simulink model "dis_lin"  (R2020b)
settings: Solver=VariableStepAuto  StartTime=0.0  StopTime=50.0  RelTol=1e-3
values from neighbouring files (symbols this model uses):
  alpha = 0.95    [main.m]
  amp = 0.3    [main.m]
  Ts = 0.15    [main.m]
  x_equ = [0.2; 0]    [main.m]
settings Model: Creator=soren  LastModifiedBy=soren

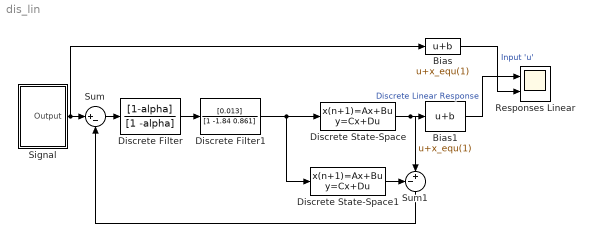
== system dis_lin ==
  Bias : Bias  Bias=x_equ(1)
  Bias1 : Bias  Bias=x_equ(1)
  Discrete Filter : DiscreteFilter  Numerator=[1-alpha]  Denominator=[1 -alpha]
  Discrete Filter1 : DiscreteFilter  Numerator=[0.013]  Denominator=[1 -1.84 0.861]
  Discrete State-Space : DiscreteStateSpace  A=[1 Ts;-3/4*Ts 1-Ts]  B=[0; 1.25*Ts]  C=[1, 0]  D=0  SampleTime=Ts
  Discrete State-Space1 : DiscreteStateSpace  A=[1 Ts;-3/4*Ts 1-Ts]  B=[0; 1.25*Ts]  C=[1, 0]  D=0  SampleTime=Ts
  Responses Linear : Scope  NumInputPorts=2
  Signal : Subsystem
  Sum : Sum  Inputs=|+-
  Sum1 : Sum  Inputs=-+|
  wires:
  Signal/1(Output) -> Bias/1, Sum/1
  Discrete Filter/1 -> Discrete Filter1/1
  Sum/1 -> Discrete Filter/1
  Discrete State-Space/1 -> Bias1/1, Sum1/2
  Discrete Filter1/1 -> Discrete State-Space1/1, Discrete State-Space/1
  Sum1/1 -> Sum/2
  Bias1/1 -> Responses Linear/1  "Discrete Linear Response"
  Bias/1 -> Responses Linear/2  "Input 'u'"
  Discrete State-Space1/1 -> Sum1/1

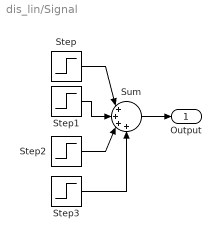
== system dis_lin/Signal ==
  Step : Step  Time=10  After=0.2*amp  SampleTime=0
  Step1 : Step  Time=20  After=-0.2*amp  SampleTime=0
  Step2 : Step  Time=30  After=-0.2*amp  SampleTime=0
  Step3 : Step  Time=40  After=0.2*amp  SampleTime=0
  Sum : Sum  Inputs=|++++
  Output : Outport
  wires:
  Sum/1 -> Output/1
  Step2/1 -> Sum/3
  Step/1 -> Sum/1
  Step1/1 -> Sum/2
  Step3/1 -> Sum/4
